simulink model "FSAC2021_V1_Running"  (R2014a)
settings: Solver=FixedStepDiscrete  StartTime=0.0  StopTime=inf  FixedStep=0.0005  RelTol=1e-3
model workspace (MAT data in the model file):
  MCOS : class17 (value not decoded)
  MCOS : class17 (value not decoded)
  MCOS : class17 (value not decoded)
  MCOS : class17 (value not decoded)
  MCOS : class17 (value not decoded)
  MCOS : class17 (value not decoded)
  MCOS : class17 (value not decoded)
  MCOS : class17 (value not decoded)
  MCOS : class17 (value not decoded)
  MCOS : class17 (value not decoded)
  MCOS : class17 (value not decoded)
  MCOS : class17 (value not decoded)
  MCOS : class17 (value not decoded)
  MCOS : class17 (value not decoded)
  MCOS : class17 (value not decoded)
  MCOS : class17 (value not decoded)
  MCOS : class17 (value not decoded)
  MCOS : class17 (value not decoded)
  MCOS : class17 (value not decoded)
  BUZZER_START = 1
  MCOS : class17 (value not decoded)
  MCOS : class17 (value not decoded)
  MCOS : class17 (value not decoded)
  MCOS : class17 (value not decoded)
  MCOS : class17 (value not decoded)
  MCOS : class17 (value not decoded)
  MCOS : class17 (value not decoded)
  MCOS : class17 (value not decoded)
  MCOS : class17 (value not decoded)
  MCOS : class17 (value not decoded)
  MCOS : class17 (value not decoded)
  MCOS : class17 (value not decoded)
  MCOS : class17 (value not decoded)
  MCOS : class17 (value not decoded)
  MCOS : class17 (value not decoded)
  MCOS : class17 (value not decoded)
  MCOS : class17 (value not decoded)
  MCOS : class17 (value not decoded)
  MCOS : class17 (value not decoded)
  MCOS : class17 (value not decoded)
  MCOS : class17 (value not decoded)
  MCOS : class17 (value not decoded)
  MCOS : class17 (value not decoded)
  MCOS : class17 (value not decoded)
  MCOS : class17 (value not decoded)
  MCOS : class17 (value not decoded)
  MCOS : class17 (value not decoded)
  MCOS : class17 (value not decoded)
  MCOS : class17 (value not decoded)
  MCOS : class17 (value not decoded)
  MCOS : class17 (value not decoded)
  MCOS : class17 (value not decoded)
  MCOS : class17 (value not decoded)
  MCOS : class17 (value not decoded)
  MCOS : class17 (value not decoded)
  MCOS : class17 (value not decoded)
  MCOS : class17 (value not decoded)
  MCOS : class17 (value not decoded)
  Brake = 11
  MCOS : class17 (value not decoded)
  MCOS : class17 (value not decoded)
  MCOS : class17 (value not decoded)
  MCOS : class17 (value not decoded)
  MCOS : class17 (value not decoded)
  MCOS : class17 (value not decoded)
  MCOS : class17 (value not decoded)
  MCOS : class17 (value not decoded)
  Sensor_Acc_b = 101.85
  Sensor_Acc_k = -0.0185
  Str_Sen_Orig_Angle = -341
  MCOS : class17 (value not decoded)
  Tire_D = 0.47
  T = 0.05
libraries: simulink x402, ec55xxlib x134
(part 11 of 17)

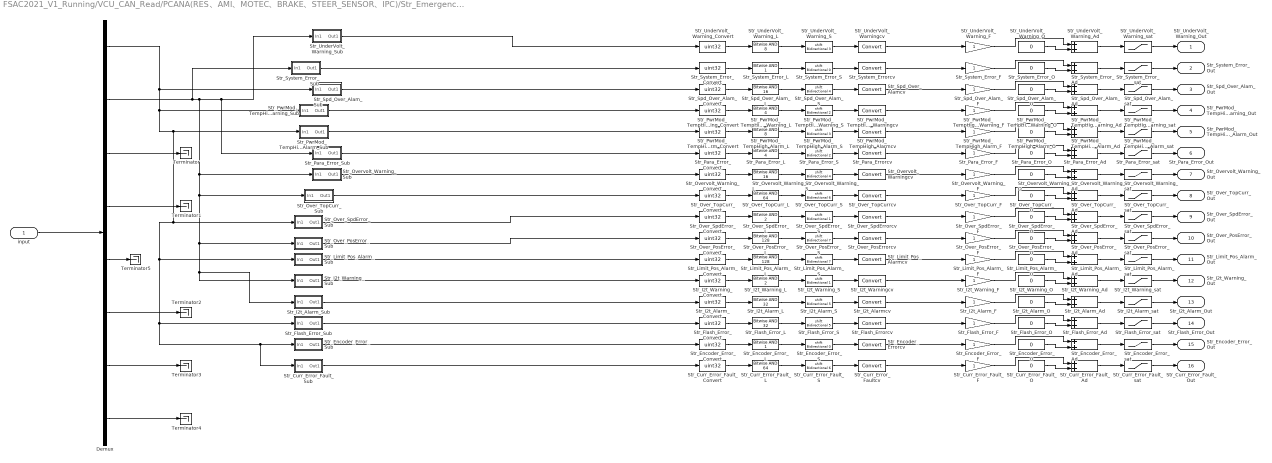
== system FSAC2021_V1_Running/VCU_CAN_Read/PCANA(RES、AMI、MOTEC、BRAKE、STEER_SENSOR、IPC)/Str_Emergency /MOTEC_EMERGENCY ==
  input : Inport
  Demux : Demux  Outputs=8
  Str_Curr_Error_Fault_Ad : Sum
  Str_Curr_Error_Fault_Convert : DataTypeConversion  OutDataTypeStr=uint32
  Str_Curr_Error_Fault_F : Gain
  Str_Curr_Error_Fault_L : simulink/Logic and Bit Operations/Bitwise Operator  logicop=AND  UseBitMask=on  BitMask=64  BitMaskRealWorld=Stored Integer
  Str_Curr_Error_Fault_O : Constant  Value=0  OutDataTypeStr=single
  Str_Curr_Error_Fault_S : ArithShift  BitShiftNumber=6
  Str_Curr_Error_Fault_Sub : Subsystem
  Str_Curr_Error_Fault_sat : Saturate  UpperLimit=1  LowerLimit=0
  Str_Curr_Error_Faultcv : DataTypeConversion
  Str_Encoder_Error_Ad : Sum
  Str_Encoder_Error_Convert : DataTypeConversion  OutDataTypeStr=uint32
  Str_Encoder_Error_F : Gain
  Str_Encoder_Error_L : simulink/Logic and Bit Operations/Bitwise Operator  logicop=AND  UseBitMask=on  BitMask=1  BitMaskRealWorld=Stored Integer
  Str_Encoder_Error_O : Constant  Value=0  OutDataTypeStr=single
  Str_Encoder_Error_S : ArithShift
  Str_Encoder_Error_Sub : Subsystem
  Str_Encoder_Error_sat : Saturate  UpperLimit=1  LowerLimit=0
  Str_Encoder_Errorcv : DataTypeConversion
  Str_Flash_Error_Ad : Sum
  Str_Flash_Error_Convert : DataTypeConversion  OutDataTypeStr=uint32
  Str_Flash_Error_F : Gain
  Str_Flash_Error_L : simulink/Logic and Bit Operations/Bitwise Operator  logicop=AND  UseBitMask=on  BitMask=32  BitMaskRealWorld=Stored Integer
  Str_Flash_Error_O : Constant  Value=0  OutDataTypeStr=single
  Str_Flash_Error_S : ArithShift  BitShiftNumber=5
  Str_Flash_Error_Sub : Subsystem
  Str_Flash_Error_sat : Saturate  UpperLimit=1  LowerLimit=0
  Str_Flash_Errorcv : DataTypeConversion
  Str_I2t_Alarm_Ad : Sum
  Str_I2t_Alarm_Convert : DataTypeConversion  OutDataTypeStr=uint32
  Str_I2t_Alarm_F : Gain
  Str_I2t_Alarm_L : simulink/Logic and Bit Operations/Bitwise Operator  logicop=AND  UseBitMask=on  BitMask=32  BitMaskRealWorld=Stored Integer
  Str_I2t_Alarm_O : Constant  Value=0  OutDataTypeStr=single
  Str_I2t_Alarm_S : ArithShift  BitShiftNumber=5
  Str_I2t_Alarm_Sub : Subsystem
  Str_I2t_Alarm_sat : Saturate  UpperLimit=1  LowerLimit=0
  Str_I2t_Alarmcv : DataTypeConversion
  Str_I2t_Warning_Ad : Sum
  Str_I2t_Warning_Convert : DataTypeConversion  OutDataTypeStr=uint32
  Str_I2t_Warning_F : Gain
  Str_I2t_Warning_L : simulink/Logic and Bit Operations/Bitwise Operator  logicop=AND  UseBitMask=on  BitMask=2  BitMaskRealWorld=Stored Integer
  Str_I2t_Warning_O : Constant  Value=0  OutDataTypeStr=single
  Str_I2t_Warning_S : ArithShift  BitShiftNumber=1
  Str_I2t_Warning_Sub : Subsystem
  Str_I2t_Warning_sat : Saturate  UpperLimit=1  LowerLimit=0
  Str_I2t_Warningcv : DataTypeConversion
  Str_Limit_Pos_Alarm_Ad : Sum
  Str_Limit_Pos_Alarm_Convert : DataTypeConversion  OutDataTypeStr=uint32
  Str_Limit_Pos_Alarm_F : Gain
  Str_Limit_Pos_Alarm_L : simulink/Logic and Bit Operations/Bitwise Operator  logicop=AND  UseBitMask=on  BitMask=128  BitMaskRealWorld=Stored Integer
  Str_Limit_Pos_Alarm_O : Constant  Value=0  OutDataTypeStr=single
  Str_Limit_Pos_Alarm_S : ArithShift  BitShiftNumber=7
  Str_Limit_Pos_Alarm_Sub : Subsystem
  Str_Limit_Pos_Alarm_sat : Saturate  UpperLimit=1  LowerLimit=0
  Str_Limit_Pos_Alarmcv : DataTypeConversion
  Str_Over_PosError_Ad : Sum
  Str_Over_PosError_Convert : DataTypeConversion  OutDataTypeStr=uint32
  Str_Over_PosError_F : Gain
  Str_Over_PosError_L : simulink/Logic and Bit Operations/Bitwise Operator  logicop=AND  UseBitMask=on  BitMask=128  BitMaskRealWorld=Stored Integer
  Str_Over_PosError_O : Constant  Value=0  OutDataTypeStr=single
  Str_Over_PosError_S : ArithShift  BitShiftNumber=7
  Str_Over_PosError_Sub : Subsystem
  Str_Over_PosError_sat : Saturate  UpperLimit=1  LowerLimit=0
  Str_Over_PosErrorcv : DataTypeConversion
  Str_Over_SpdError_Ad : Sum
  Str_Over_SpdError_Convert : DataTypeConversion  OutDataTypeStr=uint32
  Str_Over_SpdError_F : Gain
  Str_Over_SpdError_L : simulink/Logic and Bit Operations/Bitwise Operator  logicop=AND  UseBitMask=on  BitMask=2  BitMaskRealWorld=Stored Integer
  Str_Over_SpdError_O : Constant  Value=0  OutDataTypeStr=single
  Str_Over_SpdError_S : ArithShift  BitShiftNumber=1
  Str_Over_SpdError_Sub : Subsystem
  Str_Over_SpdError_sat : Saturate  UpperLimit=1  LowerLimit=0
  Str_Over_SpdErrorcv : DataTypeConversion
  Str_Over_TopCurr_Ad : Sum
  Str_Over_TopCurr_Convert : DataTypeConversion  OutDataTypeStr=uint32
  Str_Over_TopCurr_F : Gain
  Str_Over_TopCurr_L : simulink/Logic and Bit Operations/Bitwise Operator  logicop=AND  UseBitMask=on  BitMask=64  BitMaskRealWorld=Stored Integer
  Str_Over_TopCurr_O : Constant  Value=0  OutDataTypeStr=single
  Str_Over_TopCurr_S : ArithShift  BitShiftNumber=6
  Str_Over_TopCurr_Sub : Subsystem
  Str_Over_TopCurr_sat : Saturate  UpperLimit=1  LowerLimit=0
  Str_Over_TopCurrcv : DataTypeConversion
  Str_Overvolt_Warning_Ad : Sum
  Str_Overvolt_Warning_Convert : DataTypeConversion  OutDataTypeStr=uint32
  Str_Overvolt_Warning_F : Gain
  Str_Overvolt_Warning_L : simulink/Logic and Bit Operations/Bitwise Operator  logicop=AND  UseBitMask=on  BitMask=16  BitMaskRealWorld=Stored Integer
  Str_Overvolt_Warning_O : Constant  Value=0  OutDataTypeStr=single
  Str_Overvolt_Warning_S : ArithShift  BitShiftNumber=4
  Str_Overvolt_Warning_Sub : Subsystem
  Str_Overvolt_Warning_sat : Saturate  UpperLimit=1  LowerLimit=0
  Str_Overvolt_Warningcv : DataTypeConversion
  Str_Para_Error_Ad : Sum
  Str_Para_Error_Convert : DataTypeConversion  OutDataTypeStr=uint32
  Str_Para_Error_F : Gain
  Str_Para_Error_L : simulink/Logic and Bit Operations/Bitwise Operator  logicop=AND  UseBitMask=on  BitMask=4  BitMaskRealWorld=Stored Integer
  Str_Para_Error_O : Constant  Value=0  OutDataTypeStr=single
  Str_Para_Error_S : ArithShift  BitShiftNumber=2
  Str_Para_Error_Sub : Subsystem
  Str_Para_Error_sat : Saturate  UpperLimit=1  LowerLimit=0
  Str_Para_Errorcv : DataTypeConversion
  Str_PwrMod_TempHigh_Alarm_Ad : Sum
  Str_PwrMod_TempHigh_Alarm_Convert : DataTypeConversion  OutDataTypeStr=uint32
  Str_PwrMod_TempHigh_Alarm_F : Gain
  Str_PwrMod_TempHigh_Alarm_L : simulink/Logic and Bit Operations/Bitwise Operator  logicop=AND  UseBitMask=on  BitMask=8  BitMaskRealWorld=Stored Integer
  Str_PwrMod_TempHigh_Alarm_O : Constant  Value=0  OutDataTypeStr=single
  Str_PwrMod_TempHigh_Alarm_S : ArithShift  BitShiftNumber=3
  Str_PwrMod_TempHigh_Alarm_Sub : Subsystem
  Str_PwrMod_TempHigh_Alarm_sat : Saturate  UpperLimit=1  LowerLimit=0
  Str_PwrMod_TempHigh_Alarmcv : DataTypeConversion
  Str_PwrMod_TempHigh_Warning_Ad : Sum
  Str_PwrMod_TempHigh_Warning_Convert : DataTypeConversion  OutDataTypeStr=uint32
  Str_PwrMod_TempHigh_Warning_F : Gain
  Str_PwrMod_TempHigh_Warning_L : simulink/Logic and Bit Operations/Bitwise Operator  logicop=AND  UseBitMask=on  BitMask=4  BitMaskRealWorld=Stored Integer
  Str_PwrMod_TempHigh_Warning_O : Constant  Value=0  OutDataTypeStr=single
  Str_PwrMod_TempHigh_Warning_S : ArithShift  BitShiftNumber=2
  Str_PwrMod_TempHigh_Warning_Sub : Subsystem
  Str_PwrMod_TempHigh_Warning_sat : Saturate  UpperLimit=1  LowerLimit=0
  Str_PwrMod_TempHigh_Warningcv : DataTypeConversion
  Str_Spd_Over_Alam_Ad : Sum
  Str_Spd_Over_Alam_Convert : DataTypeConversion  OutDataTypeStr=uint32
  Str_Spd_Over_Alam_F : Gain
  Str_Spd_Over_Alam_L : simulink/Logic and Bit Operations/Bitwise Operator  logicop=AND  UseBitMask=on  BitMask=16  BitMaskRealWorld=Stored Integer
  Str_Spd_Over_Alam_O : Constant  Value=0  OutDataTypeStr=single
  Str_Spd_Over_Alam_S : ArithShift  BitShiftNumber=4
  Str_Spd_Over_Alam_Sub : Subsystem
  Str_Spd_Over_Alam_sat : Saturate  UpperLimit=1  LowerLimit=0
  Str_Spd_Over_Alamcv : DataTypeConversion
  Str_System_Error_Ad : Sum
  Str_System_Error_Convert : DataTypeConversion  OutDataTypeStr=uint32
  Str_System_Error_F : Gain
  Str_System_Error_L : simulink/Logic and Bit Operations/Bitwise Operator  logicop=AND  UseBitMask=on  BitMask=1  BitMaskRealWorld=Stored Integer
  Str_System_Error_O : Constant  Value=0  OutDataTypeStr=single
  Str_System_Error_S : ArithShift
  Str_System_Error_Sub : Subsystem
  Str_System_Error_sat : Saturate  UpperLimit=1  LowerLimit=0
  Str_System_Errorcv : DataTypeConversion
  Str_UnderVolt_Warning_Ad : Sum
  Str_UnderVolt_Warning_Convert : DataTypeConversion  OutDataTypeStr=uint32
  Str_UnderVolt_Warning_F : Gain
  Str_UnderVolt_Warning_L : simulink/Logic and Bit Operations/Bitwise Operator  logicop=AND  UseBitMask=on  BitMask=8  BitMaskRealWorld=Stored Integer
  Str_UnderVolt_Warning_O : Constant  Value=0  OutDataTypeStr=single
  Str_UnderVolt_Warning_S : ArithShift  BitShiftNumber=3
  Str_UnderVolt_Warning_Sub : Subsystem
  Str_UnderVolt_Warning_sat : Saturate  UpperLimit=1  LowerLimit=0
  Str_UnderVolt_Warningcv : DataTypeConversion
  Terminator{,1..5} (6 alike) : Terminator
  Str_UnderVolt_Warning_Out : Outport
  Str_System_Error_Out : Outport  Port=2
  Str_Spd_Over_Alam_Out : Outport  Port=3
  Str_PwrMod_TempHigh_Warning_Out : Outport  Port=4
  Str_PwrMod_TempHigh_Alarm_Out : Outport  Port=5
  Str_Para_Error_Out : Outport  Port=6
  Str_Overvolt_Warning_Out : Outport  Port=7
  Str_Over_TopCurr_Out : Outport  Port=8
  Str_Over_SpdError_Out : Outport  Port=9
  Str_Over_PosError_Out : Outport  Port=10
  Str_Limit_Pos_Alarm_Out : Outport  Port=11
  Str_I2t_Warning_Out : Outport  Port=12
  Str_I2t_Alarm_Out : Outport  Port=13
  Str_Flash_Error_Out : Outport  Port=14
  Str_Encoder_Error_Out : Outport  Port=15
  Str_Curr_Error_Fault_Out : Outport  Port=16
  wires:
  Str_UnderVolt_Warning_F/1 -> Str_UnderVolt_Warning_Ad/1
  Str_UnderVolt_Warning_O/1 -> Str_UnderVolt_Warning_Ad/2
  Str_UnderVolt_Warning_Ad/1 -> Str_UnderVolt_Warning_sat/1
  Str_UnderVolt_Warning_sat/1 -> Str_UnderVolt_Warning_Out/1
  Demux/2 -> Str_Para_Error_Sub/1(In1), Str_UnderVolt_Warning_Sub/1(In1), Str_I2t_Warning_Sub/1(In1), Str_I2t_Alarm_Sub/1(In1), Str_Over_PosError_Sub/1(In1), Str_Over_TopCurr_Sub/1(In1), Str_Overvolt_Warning_Sub/1(In1), Str_System_Error_Sub/1(In1)
  Str_UnderVolt_Warning_Sub/1(Out1) -> Str_UnderVolt_Warning_Convert/1
  Str_UnderVolt_Warning_Convert/1 -> Str_UnderVolt_Warning_L/1
  Str_UnderVolt_Warning_L/1 -> Str_UnderVolt_Warning_S/1
  Str_UnderVolt_Warning_S/1 -> Str_UnderVolt_Warningcv/1
  Str_UnderVolt_Warningcv/1 -> Str_UnderVolt_Warning_F/1
  Str_System_Error_F/1 -> Str_System_Error_Ad/1
  Str_System_Error_O/1 -> Str_System_Error_Ad/2
  Str_System_Error_Ad/1 -> Str_System_Error_sat/1
  Str_System_Error_sat/1 -> Str_System_Error_Out/1
  Str_System_Error_Sub/1(Out1) -> Str_System_Error_Convert/1
  Str_System_Error_Convert/1 -> Str_System_Error_L/1
  Str_System_Error_L/1 -> Str_System_Error_S/1
  Str_System_Error_S/1 -> Str_System_Errorcv/1
  Str_System_Errorcv/1 -> Str_System_Error_F/1
  Str_Spd_Over_Alam_F/1 -> Str_Spd_Over_Alam_Ad/1
  Str_Spd_Over_Alam_O/1 -> Str_Spd_Over_Alam_Ad/2
  Str_Spd_Over_Alam_Ad/1 -> Str_Spd_Over_Alam_sat/1
  Str_Spd_Over_Alam_sat/1 -> Str_Spd_Over_Alam_Out/1
  Demux/1 -> Str_Encoder_Error_Sub/1(In1), Str_Curr_Error_Fault_Sub/1(In1), Str_Flash_Error_Sub/1(In1), Str_Limit_Pos_Alarm_Sub/1(In1), Str_Over_SpdError_Sub/1(In1), Str_PwrMod_TempHigh_Alarm_Sub/1(In1), Str_PwrMod_TempHigh_Warning_Sub/1(In1), Str_Spd_Over_Alam_Sub/1(In1)
  Str_Spd_Over_Alam_Sub/1(Out1) -> Str_Spd_Over_Alam_Convert/1
  Str_Spd_Over_Alam_Convert/1 -> Str_Spd_Over_Alam_L/1
  Str_Spd_Over_Alam_L/1 -> Str_Spd_Over_Alam_S/1
  Str_Spd_Over_Alam_S/1 -> Str_Spd_Over_Alamcv/1
  Str_Spd_Over_Alamcv/1 -> Str_Spd_Over_Alam_F/1
  Str_PwrMod_TempHigh_Warning_F/1 -> Str_PwrMod_TempHigh_Warning_Ad/1
  Str_PwrMod_TempHigh_Warning_O/1 -> Str_PwrMod_TempHigh_Warning_Ad/2
  Str_PwrMod_TempHigh_Warning_Ad/1 -> Str_PwrMod_TempHigh_Warning_sat/1
  Str_PwrMod_TempHigh_Warning_sat/1 -> Str_PwrMod_TempHigh_Warning_Out/1
  Str_PwrMod_TempHigh_Warning_Sub/1(Out1) -> Str_PwrMod_TempHigh_Warning_Convert/1
  Str_PwrMod_TempHigh_Warning_Convert/1 -> Str_PwrMod_TempHigh_Warning_L/1
  Str_PwrMod_TempHigh_Warning_L/1 -> Str_PwrMod_TempHigh_Warning_S/1
  Str_PwrMod_TempHigh_Warning_S/1 -> Str_PwrMod_TempHigh_Warningcv/1
  Str_PwrMod_TempHigh_Warningcv/1 -> Str_PwrMod_TempHigh_Warning_F/1
  Str_PwrMod_TempHigh_Alarm_F/1 -> Str_PwrMod_TempHigh_Alarm_Ad/1
  Str_PwrMod_TempHigh_Alarm_O/1 -> Str_PwrMod_TempHigh_Alarm_Ad/2
  Str_PwrMod_TempHigh_Alarm_Ad/1 -> Str_PwrMod_TempHigh_Alarm_sat/1
  Str_PwrMod_TempHigh_Alarm_sat/1 -> Str_PwrMod_TempHigh_Alarm_Out/1
  Str_PwrMod_TempHigh_Alarm_Sub/1(Out1) -> Str_PwrMod_TempHigh_Alarm_Convert/1
  Str_PwrMod_TempHigh_Alarm_Convert/1 -> Str_PwrMod_TempHigh_Alarm_L/1
  Str_PwrMod_TempHigh_Alarm_L/1 -> Str_PwrMod_TempHigh_Alarm_S/1
  Str_PwrMod_TempHigh_Alarm_S/1 -> Str_PwrMod_TempHigh_Alarmcv/1
  Str_PwrMod_TempHigh_Alarmcv/1 -> Str_PwrMod_TempHigh_Alarm_F/1
  Str_Para_Error_F/1 -> Str_Para_Error_Ad/1
  Str_Para_Error_O/1 -> Str_Para_Error_Ad/2
  Str_Para_Error_Ad/1 -> Str_Para_Error_sat/1
  Str_Para_Error_sat/1 -> Str_Para_Error_Out/1
  Str_Para_Error_Sub/1(Out1) -> Str_Para_Error_Convert/1
  Str_Para_Error_Convert/1 -> Str_Para_Error_L/1
  Str_Para_Error_L/1 -> Str_Para_Error_S/1
  Str_Para_Error_S/1 -> Str_Para_Errorcv/1
  Str_Para_Errorcv/1 -> Str_Para_Error_F/1
  Str_Overvolt_Warning_F/1 -> Str_Overvolt_Warning_Ad/1
  Str_Overvolt_Warning_O/1 -> Str_Overvolt_Warning_Ad/2
  Str_Overvolt_Warning_Ad/1 -> Str_Overvolt_Warning_sat/1
  Str_Overvolt_Warning_sat/1 -> Str_Overvolt_Warning_Out/1
  Str_Overvolt_Warning_Sub/1(Out1) -> Str_Overvolt_Warning_Convert/1
  Str_Overvolt_Warning_Convert/1 -> Str_Overvolt_Warning_L/1
  Str_Overvolt_Warning_L/1 -> Str_Overvolt_Warning_S/1
  Str_Overvolt_Warning_S/1 -> Str_Overvolt_Warningcv/1
  Str_Overvolt_Warningcv/1 -> Str_Overvolt_Warning_F/1
  Str_Over_TopCurr_F/1 -> Str_Over_TopCurr_Ad/1
  Str_Over_TopCurr_O/1 -> Str_Over_TopCurr_Ad/2
  Str_Over_TopCurr_Ad/1 -> Str_Over_TopCurr_sat/1
  Str_Over_TopCurr_sat/1 -> Str_Over_TopCurr_Out/1
  Str_Over_TopCurr_Sub/1(Out1) -> Str_Over_TopCurr_Convert/1
  Str_Over_TopCurr_Convert/1 -> Str_Over_TopCurr_L/1
  Str_Over_TopCurr_L/1 -> Str_Over_TopCurr_S/1
  Str_Over_TopCurr_S/1 -> Str_Over_TopCurrcv/1
  Str_Over_TopCurrcv/1 -> Str_Over_TopCurr_F/1
  Str_Over_SpdError_F/1 -> Str_Over_SpdError_Ad/1
  Str_Over_SpdError_O/1 -> Str_Over_SpdError_Ad/2
  Str_Over_SpdError_Ad/1 -> Str_Over_SpdError_sat/1
  Str_Over_SpdError_sat/1 -> Str_Over_SpdError_Out/1
  Str_Over_SpdError_Sub/1(Out1) -> Str_Over_SpdError_Convert/1
  Str_Over_SpdError_Convert/1 -> Str_Over_SpdError_L/1
  Str_Over_SpdError_L/1 -> Str_Over_SpdError_S/1
  Str_Over_SpdError_S/1 -> Str_Over_SpdErrorcv/1
  Str_Over_SpdErrorcv/1 -> Str_Over_SpdError_F/1
  Str_Over_PosError_F/1 -> Str_Over_PosError_Ad/1
  Str_Over_PosError_O/1 -> Str_Over_PosError_Ad/2
  Str_Over_PosError_Ad/1 -> Str_Over_PosError_sat/1
  Str_Over_PosError_sat/1 -> Str_Over_PosError_Out/1
  Str_Over_PosError_Sub/1(Out1) -> Str_Over_PosError_Convert/1
  Str_Over_PosError_Convert/1 -> Str_Over_PosError_L/1
  Str_Over_PosError_L/1 -> Str_Over_PosError_S/1
  Str_Over_PosError_S/1 -> Str_Over_PosErrorcv/1
  Str_Over_PosErrorcv/1 -> Str_Over_PosError_F/1
  Str_Limit_Pos_Alarm_F/1 -> Str_Limit_Pos_Alarm_Ad/1
  Str_Limit_Pos_Alarm_O/1 -> Str_Limit_Pos_Alarm_Ad/2
  Str_Limit_Pos_Alarm_Ad/1 -> Str_Limit_Pos_Alarm_sat/1
  Str_Limit_Pos_Alarm_sat/1 -> Str_Limit_Pos_Alarm_Out/1
  Str_Limit_Pos_Alarm_Sub/1(Out1) -> Str_Limit_Pos_Alarm_Convert/1
  Str_Limit_Pos_Alarm_Convert/1 -> Str_Limit_Pos_Alarm_L/1
  Str_Limit_Pos_Alarm_L/1 -> Str_Limit_Pos_Alarm_S/1
  Str_Limit_Pos_Alarm_S/1 -> Str_Limit_Pos_Alarmcv/1
  Str_Limit_Pos_Alarmcv/1 -> Str_Limit_Pos_Alarm_F/1
  Str_I2t_Warning_F/1 -> Str_I2t_Warning_Ad/1
  Str_I2t_Warning_O/1 -> Str_I2t_Warning_Ad/2
  Str_I2t_Warning_Ad/1 -> Str_I2t_Warning_sat/1
  Str_I2t_Warning_sat/1 -> Str_I2t_Warning_Out/1
  Str_I2t_Warning_Sub/1(Out1) -> Str_I2t_Warning_Convert/1
  Str_I2t_Warning_Convert/1 -> Str_I2t_Warning_L/1
  Str_I2t_Warning_L/1 -> Str_I2t_Warning_S/1
  Str_I2t_Warning_S/1 -> Str_I2t_Warningcv/1
  Str_I2t_Warningcv/1 -> Str_I2t_Warning_F/1
  Str_I2t_Alarm_F/1 -> Str_I2t_Alarm_Ad/1
  Str_I2t_Alarm_O/1 -> Str_I2t_Alarm_Ad/2
  Str_I2t_Alarm_Ad/1 -> Str_I2t_Alarm_sat/1
  Str_I2t_Alarm_sat/1 -> Str_I2t_Alarm_Out/1
  Str_I2t_Alarm_Sub/1(Out1) -> Str_I2t_Alarm_Convert/1
  Str_I2t_Alarm_Convert/1 -> Str_I2t_Alarm_L/1
  Str_I2t_Alarm_L/1 -> Str_I2t_Alarm_S/1
  Str_I2t_Alarm_S/1 -> Str_I2t_Alarmcv/1
  Str_I2t_Alarmcv/1 -> Str_I2t_Alarm_F/1
  Str_Flash_Error_F/1 -> Str_Flash_Error_Ad/1
  Str_Flash_Error_O/1 -> Str_Flash_Error_Ad/2
  Str_Flash_Error_Ad/1 -> Str_Flash_Error_sat/1
  Str_Flash_Error_sat/1 -> Str_Flash_Error_Out/1
  Str_Flash_Error_Sub/1(Out1) -> Str_Flash_Error_Convert/1
  Str_Flash_Error_Convert/1 -> Str_Flash_Error_L/1
  Str_Flash_Error_L/1 -> Str_Flash_Error_S/1
  Str_Flash_Error_S/1 -> Str_Flash_Errorcv/1
  Str_Flash_Errorcv/1 -> Str_Flash_Error_F/1
  Str_Encoder_Error_F/1 -> Str_Encoder_Error_Ad/1
  Str_Encoder_Error_O/1 -> Str_Encoder_Error_Ad/2
  Str_Encoder_Error_Ad/1 -> Str_Encoder_Error_sat/1
  Str_Encoder_Error_sat/1 -> Str_Encoder_Error_Out/1
  Str_Encoder_Error_Sub/1(Out1) -> Str_Encoder_Error_Convert/1
  Str_Encoder_Error_Convert/1 -> Str_Encoder_Error_L/1
  Str_Encoder_Error_L/1 -> Str_Encoder_Error_S/1
  Str_Encoder_Error_S/1 -> Str_Encoder_Errorcv/1
  Str_Encoder_Errorcv/1 -> Str_Encoder_Error_F/1
  Str_Curr_Error_Fault_F/1 -> Str_Curr_Error_Fault_Ad/1
  Str_Curr_Error_Fault_O/1 -> Str_Curr_Error_Fault_Ad/2
  Str_Curr_Error_Fault_Ad/1 -> Str_Curr_Error_Fault_sat/1
  Str_Curr_Error_Fault_sat/1 -> Str_Curr_Error_Fault_Out/1
  Str_Curr_Error_Fault_Sub/1(Out1) -> Str_Curr_Error_Fault_Convert/1
  Str_Curr_Error_Fault_Convert/1 -> Str_Curr_Error_Fault_L/1
  Str_Curr_Error_Fault_L/1 -> Str_Curr_Error_Fault_S/1
  Str_Curr_Error_Fault_S/1 -> Str_Curr_Error_Faultcv/1
  Str_Curr_Error_Faultcv/1 -> Str_Curr_Error_Fault_F/1
  input/1 -> Demux/1
  Demux/3 -> Terminator/1
  Demux/4 -> Terminator1/1
  Demux/6 -> Terminator2/1
  Demux/7 -> Terminator3/1
  Demux/8 -> Terminator4/1
  Demux/5 -> Terminator5/1

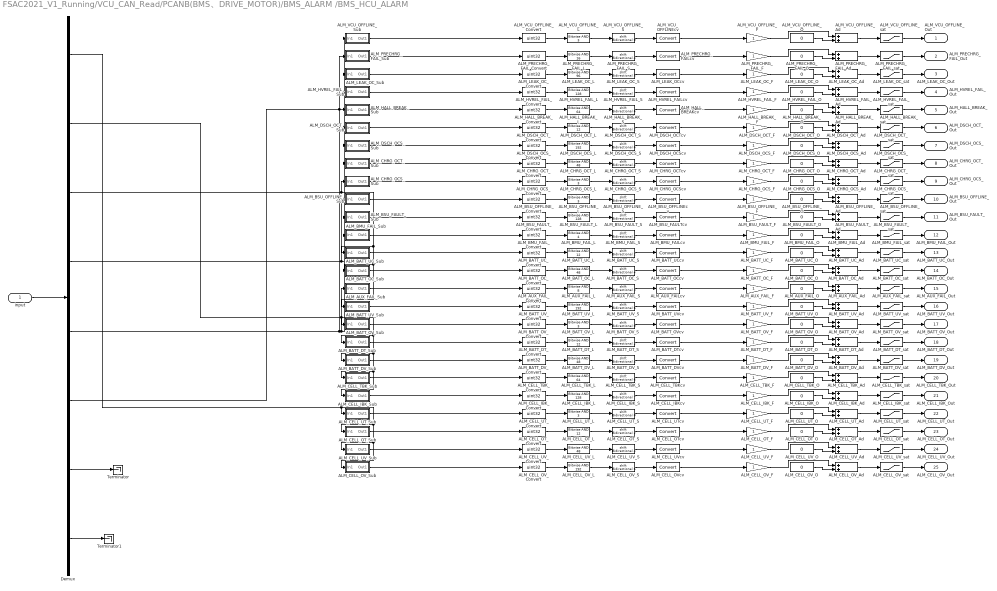
== system FSAC2021_V1_Running/VCU_CAN_Read/PCANB(BMS、DRIVE_MOTOR)/BMS_ALARM /BMS_HCU_ALARM ==
  input : Inport
  ALM_AUX_FAIL_Ad : Sum
  ALM_AUX_FAIL_Convert : DataTypeConversion  OutDataTypeStr=uint32
  ALM_AUX_FAIL_F : Gain
  ALM_AUX_FAIL_L : simulink/Logic and Bit Operations/Bitwise Operator  logicop=AND  UseBitMask=on  BitMask=8  BitMaskRealWorld=Stored Integer
  ALM_AUX_FAIL_O : Constant  Value=0  OutDataTypeStr=single
  ALM_AUX_FAIL_S : ArithShift  BitShiftNumber=3
  ALM_AUX_FAIL_Sub : Subsystem
  ALM_AUX_FAIL_sat : Saturate  UpperLimit=1  LowerLimit=0
  ALM_AUX_FAILcv : DataTypeConversion
  ALM_BATT_DT_Ad : Sum
  ALM_BATT_DT_Convert : DataTypeConversion  OutDataTypeStr=uint32
  ALM_BATT_DT_F : Gain
  ALM_BATT_DT_L : simulink/Logic and Bit Operations/Bitwise Operator  logicop=AND  UseBitMask=on  BitMask=12  BitMaskRealWorld=Stored Integer
  ALM_BATT_DT_O : Constant  Value=0  OutDataTypeStr=single
  ALM_BATT_DT_S : ArithShift  BitShiftNumber=2
  ALM_BATT_DT_Sub : Subsystem
  ALM_BATT_DT_sat : Saturate  UpperLimit=3  LowerLimit=0
  ALM_BATT_DTcv : DataTypeConversion
  ALM_BATT_DV_Ad : Sum
  ALM_BATT_DV_Convert : DataTypeConversion  OutDataTypeStr=uint32
  ALM_BATT_DV_F : Gain
  ALM_BATT_DV_L : simulink/Logic and Bit Operations/Bitwise Operator  logicop=AND  UseBitMask=on  BitMask=48  BitMaskRealWorld=Stored Integer
  ALM_BATT_DV_O : Constant  Value=0  OutDataTypeStr=single
  ALM_BATT_DV_S : ArithShift  BitShiftNumber=4
  ALM_BATT_DV_Sub : Subsystem
  ALM_BATT_DV_sat : Saturate  UpperLimit=3  LowerLimit=0
  ALM_BATT_DVcv : DataTypeConversion
  ALM_BATT_OC_Ad : Sum
  ALM_BATT_OC_Convert : DataTypeConversion  OutDataTypeStr=uint32
  ALM_BATT_OC_F : Gain
  ALM_BATT_OC_L : simulink/Logic and Bit Operations/Bitwise Operator  logicop=AND  UseBitMask=on  BitMask=48  BitMaskRealWorld=Stored Integer
  ALM_BATT_OC_O : Constant  Value=0  OutDataTypeStr=single
  ALM_BATT_OC_S : ArithShift  BitShiftNumber=4
  ALM_BATT_OC_Sub : Subsystem
  ALM_BATT_OC_sat : Saturate  UpperLimit=3  LowerLimit=0
  ALM_BATT_OCcv : DataTypeConversion
  ALM_BATT_OV_Ad : Sum
  ALM_BATT_OV_Convert : DataTypeConversion  OutDataTypeStr=uint32
  ALM_BATT_OV_F : Gain
  ALM_BATT_OV_L : simulink/Logic and Bit Operations/Bitwise Operator  logicop=AND  UseBitMask=on  BitMask=3  BitMaskRealWorld=Stored Integer
  ALM_BATT_OV_O : Constant  Value=0  OutDataTypeStr=single
  ALM_BATT_OV_S : ArithShift
  ALM_BATT_OV_Sub : Subsystem
  ALM_BATT_OV_sat : Saturate  UpperLimit=3  LowerLimit=0
  ALM_BATT_OVcv : DataTypeConversion
  ALM_BATT_UC_Ad : Sum
  ALM_BATT_UC_Convert : DataTypeConversion  OutDataTypeStr=uint32
  ALM_BATT_UC_F : Gain
  ALM_BATT_UC_L : simulink/Logic and Bit Operations/Bitwise Operator  logicop=AND  UseBitMask=on  BitMask=12  BitMaskRealWorld=Stored Integer
  ALM_BATT_UC_O : Constant  Value=0  OutDataTypeStr=single
  ALM_BATT_UC_S : ArithShift  BitShiftNumber=2
  ALM_BATT_UC_Sub : Subsystem
  ALM_BATT_UC_sat : Saturate  UpperLimit=3  LowerLimit=0
  ALM_BATT_UCcv : DataTypeConversion
  ALM_BATT_UV_Ad : Sum
  ALM_BATT_UV_Convert : DataTypeConversion  OutDataTypeStr=uint32
  ALM_BATT_UV_F : Gain
  ALM_BATT_UV_L : simulink/Logic and Bit Operations/Bitwise Operator  logicop=AND  UseBitMask=on  BitMask=192  BitMaskRealWorld=Stored Integer
  ALM_BATT_UV_O : Constant  Value=0  OutDataTypeStr=single
  ALM_BATT_UV_S : ArithShift  BitShiftNumber=6
  ALM_BATT_UV_Sub : Subsystem
  ALM_BATT_UV_sat : Saturate  UpperLimit=3  LowerLimit=0
  ALM_BATT_UVcv : DataTypeConversion
  ALM_BMU_FAIL_Ad : Sum
  ALM_BMU_FAIL_Convert : DataTypeConversion  OutDataTypeStr=uint32
  ALM_BMU_FAIL_F : Gain
  ALM_BMU_FAIL_L : simulink/Logic and Bit Operations/Bitwise Operator  logicop=AND  UseBitMask=on  BitMask=4  BitMaskRealWorld=Stored Integer
  ALM_BMU_FAIL_O : Constant  Value=0  OutDataTypeStr=single
  ALM_BMU_FAIL_S : ArithShift  BitShiftNumber=2
  ALM_BMU_FAIL_Sub : Subsystem
  ALM_BMU_FAIL_sat : Saturate  UpperLimit=1  LowerLimit=0
  ALM_BMU_FAILcv : DataTypeConversion
  ALM_BSU_FAULT_Ad : Sum
  ALM_BSU_FAULT_Convert : DataTypeConversion  OutDataTypeStr=uint32
  ALM_BSU_FAULT_F : Gain
  ALM_BSU_FAULT_L : simulink/Logic and Bit Operations/Bitwise Operator  logicop=AND  UseBitMask=on  BitMask=128  BitMaskRealWorld=Stored Integer
  ALM_BSU_FAULT_O : Constant  Value=0  OutDataTypeStr=single
  ALM_BSU_FAULT_S : ArithShift  BitShiftNumber=7
  ALM_BSU_FAULT_Sub : Subsystem
  ALM_BSU_FAULT_sat : Saturate  UpperLimit=1  LowerLimit=0
  ALM_BSU_FAULTcv : DataTypeConversion
  ALM_BSU_OFFLINE_Ad : Sum
  ALM_BSU_OFFLINE_Convert : DataTypeConversion  OutDataTypeStr=uint32
  ALM_BSU_OFFLINE_F : Gain
  ALM_BSU_OFFLINE_L : simulink/Logic and Bit Operations/Bitwise Operator  logicop=AND  UseBitMask=on  BitMask=3  BitMaskRealWorld=Stored Integer
  ALM_BSU_OFFLINE_O : Constant  Value=0  OutDataTypeStr=single
  ALM_BSU_OFFLINE_S : ArithShift
  ALM_BSU_OFFLINE_Sub : Subsystem
  ALM_BSU_OFFLINE_sat : Saturate  UpperLimit=3  LowerLimit=0
  ALM_BSU_OFFLINEcv : DataTypeConversion
  ALM_CELL_IBK_Ad : Sum
  ALM_CELL_IBK_Convert : DataTypeConversion  OutDataTypeStr=uint32
  ALM_CELL_IBK_F : Gain
  ALM_CELL_IBK_L : simulink/Logic and Bit Operations/Bitwise Operator  logicop=AND  UseBitMask=on  BitMask=128  BitMaskRealWorld=Stored Integer
  ALM_CELL_IBK_O : Constant  Value=0  OutDataTypeStr=single
  ALM_CELL_IBK_S : ArithShift  BitShiftNumber=7
  ALM_CELL_IBK_Sub : Subsystem
  ALM_CELL_IBK_sat : Saturate  UpperLimit=1  LowerLimit=0
  ALM_CELL_IBKcv : DataTypeConversion
  ALM_CELL_OT_Ad : Sum
  ALM_CELL_OT_Convert : DataTypeConversion  OutDataTypeStr=uint32
  ALM_CELL_OT_F : Gain
  ALM_CELL_OT_L : simulink/Logic and Bit Operations/Bitwise Operator  logicop=AND  UseBitMask=on  BitMask=12  BitMaskRealWorld=Stored Integer
  ALM_CELL_OT_O : Constant  Value=0  OutDataTypeStr=single
  ALM_CELL_OT_S : ArithShift  BitShiftNumber=2
  ALM_CELL_OT_Sub : Subsystem
  ALM_CELL_OT_sat : Saturate  UpperLimit=3  LowerLimit=0
  ALM_CELL_OTcv : DataTypeConversion
  ALM_CELL_OV_Ad : Sum
  ALM_CELL_OV_Convert : DataTypeConversion  OutDataTypeStr=uint32
  ALM_CELL_OV_F : Gain
  ALM_CELL_OV_L : simulink/Logic and Bit Operations/Bitwise Operator  logicop=AND  UseBitMask=on  BitMask=192  BitMaskRealWorld=Stored Integer
  ALM_CELL_OV_O : Constant  Value=0  OutDataTypeStr=single
  ALM_CELL_OV_S : ArithShift  BitShiftNumber=6
  ALM_CELL_OV_Sub : Subsystem
  ALM_CELL_OV_sat : Saturate  UpperLimit=3  LowerLimit=0
  ALM_CELL_OVcv : DataTypeConversion
  ALM_CELL_TBK_Ad : Sum
  ALM_CELL_TBK_Convert : DataTypeConversion  OutDataTypeStr=uint32
  ALM_CELL_TBK_F : Gain
  ALM_CELL_TBK_L : simulink/Logic and Bit Operations/Bitwise Operator  logicop=AND  UseBitMask=on  BitMask=64  BitMaskRealWorld=Stored Integer
  ALM_CELL_TBK_O : Constant  Value=0  OutDataTypeStr=single
  ALM_CELL_TBK_S : ArithShift  BitShiftNumber=6
  ALM_CELL_TBK_Sub : Subsystem
  ALM_CELL_TBK_sat : Saturate  UpperLimit=1  LowerLimit=0
  ALM_CELL_TBKcv : DataTypeConversion
  ALM_CELL_UT_Ad : Sum
  ALM_CELL_UT_Convert : DataTypeConversion  OutDataTypeStr=uint32
  ALM_CELL_UT_F : Gain
  ALM_CELL_UT_L : simulink/Logic and Bit Operations/Bitwise Operator  logicop=AND  UseBitMask=on  BitMask=3  BitMaskRealWorld=Stored Integer
  ALM_CELL_UT_O : Constant  Value=0  OutDataTypeStr=single
  ALM_CELL_UT_S : ArithShift
  ALM_CELL_UT_Sub : Subsystem
  ALM_CELL_UT_sat : Saturate  UpperLimit=3  LowerLimit=0
  ALM_CELL_UTcv : DataTypeConversion
  ALM_CELL_UV_Ad : Sum
  ALM_CELL_UV_Convert : DataTypeConversion  OutDataTypeStr=uint32
  ALM_CELL_UV_F : Gain
  ALM_CELL_UV_L : simulink/Logic and Bit Operations/Bitwise Operator  logicop=AND  UseBitMask=on  BitMask=48  BitMaskRealWorld=Stored Integer
  ALM_CELL_UV_O : Constant  Value=0  OutDataTypeStr=single
  ALM_CELL_UV_S : ArithShift  BitShiftNumber=4
  ALM_CELL_UV_Sub : Subsystem
  ALM_CELL_UV_sat : Saturate  UpperLimit=3  LowerLimit=0
  ALM_CELL_UVcv : DataTypeConversion
  ALM_CHRG_OCS_Ad : Sum
  ALM_CHRG_OCS_Convert : DataTypeConversion  OutDataTypeStr=uint32
  ALM_CHRG_OCS_F : Gain
  ALM_CHRG_OCS_L : simulink/Logic and Bit Operations/Bitwise Operator  logicop=AND  UseBitMask=on  BitMask=3  BitMaskRealWorld=Stored Integer
  ALM_CHRG_OCS_O : Constant  Value=0  OutDataTypeStr=single
  ALM_CHRG_OCS_S : ArithShift
  ALM_CHRG_OCS_Sub : Subsystem
  ALM_CHRG_OCS_sat : Saturate  UpperLimit=3  LowerLimit=0
  ALM_CHRG_OCScv : DataTypeConversion
  ALM_CHRG_OCT_Ad : Sum
  ALM_CHRG_OCT_Convert : DataTypeConversion  OutDataTypeStr=uint32
  ALM_CHRG_OCT_F : Gain
  ALM_CHRG_OCT_L : simulink/Logic and Bit Operations/Bitwise Operator  logicop=AND  UseBitMask=on  BitMask=48  BitMaskRealWorld=Stored Integer
  ALM_CHRG_OCT_O : Constant  Value=0  OutDataTypeStr=single
  ALM_CHRG_OCT_S : ArithShift  BitShiftNumber=4
  ALM_CHRG_OCT_Sub : Subsystem
  ALM_CHRG_OCT_sat : Saturate  UpperLimit=3  LowerLimit=0
  ALM_CHRG_OCTcv : DataTypeConversion
  ALM_DSCH_OCS_Ad : Sum
  ALM_DSCH_OCS_Convert : DataTypeConversion  OutDataTypeStr=uint32
  ALM_DSCH_OCS_F : Gain
  ALM_DSCH_OCS_L : simulink/Logic and Bit Operations/Bitwise Operator  logicop=AND  UseBitMask=on  BitMask=192  BitMaskRealWorld=Stored Integer
  ALM_DSCH_OCS_O : Constant  Value=0  OutDataTypeStr=single
  ALM_DSCH_OCS_S : ArithShift  BitShiftNumber=6
  ALM_DSCH_OCS_Sub : Subsystem
  ALM_DSCH_OCS_sat : Saturate  UpperLimit=3  LowerLimit=0
  ALM_DSCH_OCScv : DataTypeConversion
  ALM_DSCH_OCT_Ad : Sum
  ALM_DSCH_OCT_Convert : DataTypeConversion  OutDataTypeStr=uint32
  ALM_DSCH_OCT_F : Gain
  ALM_DSCH_OCT_L : simulink/Logic and Bit Operations/Bitwise Operator  logicop=AND  UseBitMask=on  BitMask=12  BitMaskRealWorld=Stored Integer
  ALM_DSCH_OCT_O : Constant  Value=0  OutDataTypeStr=single
  ALM_DSCH_OCT_S : ArithShift  BitShiftNumber=2
  ALM_DSCH_OCT_Sub : Subsystem
  ALM_DSCH_OCT_sat : Saturate  UpperLimit=3  LowerLimit=0
  ALM_DSCH_OCTcv : DataTypeConversion
  ALM_HALL_BREAK_Ad : Sum
  ALM_HALL_BREAK_Convert : DataTypeConversion  OutDataTypeStr=uint32
  ALM_HALL_BREAK_F : Gain
  ALM_HALL_BREAK_L : simulink/Logic and Bit Operations/Bitwise Operator  logicop=AND  UseBitMask=on  BitMask=64  BitMaskRealWorld=Stored Integer
  ALM_HALL_BREAK_O : Constant  Value=0  OutDataTypeStr=single
  ALM_HALL_BREAK_S : ArithShift  BitShiftNumber=6
  ALM_HALL_BREAK_Sub : Subsystem
  ALM_HALL_BREAK_sat : Saturate  UpperLimit=1  LowerLimit=0
  ALM_HALL_BREAKcv : DataTypeConversion
  ALM_HVREL_FAIL_Ad : Sum
  ALM_HVREL_FAIL_Convert : DataTypeConversion  OutDataTypeStr=uint32
  ALM_HVREL_FAIL_F : Gain
  ALM_HVREL_FAIL_L : simulink/Logic and Bit Operations/Bitwise Operator  logicop=AND  UseBitMask=on  BitMask=128  BitMaskRealWorld=Stored Integer
  ALM_HVREL_FAIL_O : Constant  Value=0  OutDataTypeStr=single
  ALM_HVREL_FAIL_S : ArithShift  BitShiftNumber=7
  ALM_HVREL_FAIL_Sub : Subsystem
  ALM_HVREL_FAIL_sat : Saturate  UpperLimit=1  LowerLimit=0
  ALM_HVREL_FAILcv : DataTypeConversion
  ALM_LEAK_OC_Ad : Sum
  ALM_LEAK_OC_Convert : DataTypeConversion  OutDataTypeStr=uint32
  ALM_LEAK_OC_F : Gain
  ALM_LEAK_OC_L : simulink/Logic and Bit Operations/Bitwise Operator  logicop=AND  UseBitMask=on  BitMask=96  BitMaskRealWorld=Stored Integer
  ALM_LEAK_OC_O : Constant  Value=0  OutDataTypeStr=single
  ALM_LEAK_OC_S : ArithShift  BitShiftNumber=5
  ALM_LEAK_OC_Sub : Subsystem
  ALM_LEAK_OC_sat : Saturate  UpperLimit=3  LowerLimit=0
  ALM_LEAK_OCcv : DataTypeConversion
  ALM_PRECHRG_FAIL_Ad : Sum
  ALM_PRECHRG_FAIL_Convert : DataTypeConversion  OutDataTypeStr=uint32
  ALM_PRECHRG_FAIL_F : Gain
  ALM_PRECHRG_FAIL_L : simulink/Logic and Bit Operations/Bitwise Operator  logicop=AND  UseBitMask=on  BitMask=16  BitMaskRealWorld=Stored Integer
  ALM_PRECHRG_FAIL_O : Constant  Value=0  OutDataTypeStr=single
  ALM_PRECHRG_FAIL_S : ArithShift  BitShiftNumber=4
  ALM_PRECHRG_FAIL_Sub : Subsystem
  ALM_PRECHRG_FAIL_sat : Saturate  UpperLimit=1  LowerLimit=0
  ALM_PRECHRG_FAILcv : DataTypeConversion
  ALM_VCU_OFFLINE_Ad : Sum
  ALM_VCU_OFFLINE_Convert : DataTypeConversion  OutDataTypeStr=uint32
  ALM_VCU_OFFLINE_F : Gain
  ALM_VCU_OFFLINE_L : simulink/Logic and Bit Operations/Bitwise Operator  logicop=AND  UseBitMask=on  BitMask=3  BitMaskRealWorld=Stored Integer
  ALM_VCU_OFFLINE_O : Constant  Value=0  OutDataTypeStr=single
  ALM_VCU_OFFLINE_S : ArithShift
  ALM_VCU_OFFLINE_Sub : Subsystem
  ALM_VCU_OFFLINE_sat : Saturate  UpperLimit=3  LowerLimit=0
  ALM_VCU_OFFLINEcv : DataTypeConversion
  Demux : Demux  Outputs=8
  Terminator : Terminator
  Terminator1 : Terminator
  ALM_VCU_OFFLINE_Out : Outport
  ALM_PRECHRG_FAIL_Out : Outport  Port=2
  ALM_LEAK_OC_Out : Outport  Port=3
  ALM_HVREL_FAIL_Out : Outport  Port=4
  ALM_HALL_BREAK_Out : Outport  Port=5
  ALM_DSCH_OCT_Out : Outport  Port=6
  ALM_DSCH_OCS_Out : Outport  Port=7
  ALM_CHRG_OCT_Out : Outport  Port=8
  ALM_CHRG_OCS_Out : Outport  Port=9
  ALM_BSU_OFFLINE_Out : Outport  Port=10
  ALM_BSU_FAULT_Out : Outport  Port=11
  ALM_BMU_FAIL_Out : Outport  Port=12
  ALM_BATT_UC_Out : Outport  Port=13
  ALM_BATT_OC_Out : Outport  Port=14
  ALM_AUX_FAIL_Out : Outport  Port=15
  ALM_BATT_UV_Out : Outport  Port=16
  ALM_BATT_OV_Out : Outport  Port=17
  ALM_BATT_DT_Out : Outport  Port=18
  ALM_BATT_DV_Out : Outport  Port=19
  ALM_CELL_TBK_Out : Outport  Port=20
  ALM_CELL_IBK_Out : Outport  Port=21
  ALM_CELL_UT_Out : Outport  Port=22
  ALM_CELL_OT_Out : Outport  Port=23
  ALM_CELL_UV_Out : Outport  Port=24
  ALM_CELL_OV_Out : Outport  Port=25
  wires:
  ALM_VCU_OFFLINE_F/1 -> ALM_VCU_OFFLINE_Ad/1
  ALM_VCU_OFFLINE_O/1 -> ALM_VCU_OFFLINE_Ad/2
  ALM_VCU_OFFLINE_Ad/1 -> ALM_VCU_OFFLINE_sat/1
  ALM_VCU_OFFLINE_sat/1 -> ALM_VCU_OFFLINE_Out/1
  Demux/5 -> ALM_VCU_OFFLINE_Sub/1(In1), ALM_LEAK_OC_Sub/1(In1), ALM_BSU_FAULT_Sub/1(In1), ALM_BMU_FAIL_Sub/1(In1), ALM_AUX_FAIL_Sub/1(In1), ALM_PRECHRG_FAIL_Sub/1(In1)
  ALM_VCU_OFFLINE_Sub/1(Out1) -> ALM_VCU_OFFLINE_Convert/1
  ALM_VCU_OFFLINE_Convert/1 -> ALM_VCU_OFFLINE_L/1
  ALM_VCU_OFFLINE_L/1 -> ALM_VCU_OFFLINE_S/1
  ALM_VCU_OFFLINE_S/1 -> ALM_VCU_OFFLINEcv/1
  ALM_VCU_OFFLINEcv/1 -> ALM_VCU_OFFLINE_F/1
  ALM_PRECHRG_FAIL_F/1 -> ALM_PRECHRG_FAIL_Ad/1
  ALM_PRECHRG_FAIL_O/1 -> ALM_PRECHRG_FAIL_Ad/2
  ALM_PRECHRG_FAIL_Ad/1 -> ALM_PRECHRG_FAIL_sat/1
  ALM_PRECHRG_FAIL_sat/1 -> ALM_PRECHRG_FAIL_Out/1
  ALM_PRECHRG_FAIL_Sub/1(Out1) -> ALM_PRECHRG_FAIL_Convert/1
  ALM_PRECHRG_FAIL_Convert/1 -> ALM_PRECHRG_FAIL_L/1
  ALM_PRECHRG_FAIL_L/1 -> ALM_PRECHRG_FAIL_S/1
  ALM_PRECHRG_FAIL_S/1 -> ALM_PRECHRG_FAILcv/1
  ALM_PRECHRG_FAILcv/1 -> ALM_PRECHRG_FAIL_F/1
  ALM_LEAK_OC_F/1 -> ALM_LEAK_OC_Ad/1
  ALM_LEAK_OC_O/1 -> ALM_LEAK_OC_Ad/2
  ALM_LEAK_OC_Ad/1 -> ALM_LEAK_OC_sat/1
  ALM_LEAK_OC_sat/1 -> ALM_LEAK_OC_Out/1
  ALM_LEAK_OC_Sub/1(Out1) -> ALM_LEAK_OC_Convert/1
  ALM_LEAK_OC_Convert/1 -> ALM_LEAK_OC_L/1
  ALM_LEAK_OC_L/1 -> ALM_LEAK_OC_S/1
  ALM_LEAK_OC_S/1 -> ALM_LEAK_OCcv/1
  ALM_LEAK_OCcv/1 -> ALM_LEAK_OC_F/1
  ALM_HVREL_FAIL_F/1 -> ALM_HVREL_FAIL_Ad/1
  ALM_HVREL_FAIL_O/1 -> ALM_HVREL_FAIL_Ad/2
  ALM_HVREL_FAIL_Ad/1 -> ALM_HVREL_FAIL_sat/1
  ALM_HVREL_FAIL_sat/1 -> ALM_HVREL_FAIL_Out/1
  Demux/6 -> ALM_HVREL_FAIL_Sub/1(In1), ALM_HALL_BREAK_Sub/1(In1)
  ALM_HVREL_FAIL_Sub/1(Out1) -> ALM_HVREL_FAIL_Convert/1
  ALM_HVREL_FAIL_Convert/1 -> ALM_HVREL_FAIL_L/1
  ALM_HVREL_FAIL_L/1 -> ALM_HVREL_FAIL_S/1
  ALM_HVREL_FAIL_S/1 -> ALM_HVREL_FAILcv/1
  ALM_HVREL_FAILcv/1 -> ALM_HVREL_FAIL_F/1
  ALM_HALL_BREAK_F/1 -> ALM_HALL_BREAK_Ad/1
  ALM_HALL_BREAK_O/1 -> ALM_HALL_BREAK_Ad/2
  ALM_HALL_BREAK_Ad/1 -> ALM_HALL_BREAK_sat/1
  ALM_HALL_BREAK_sat/1 -> ALM_HALL_BREAK_Out/1
  ALM_HALL_BREAK_Sub/1(Out1) -> ALM_HALL_BREAK_Convert/1
  ALM_HALL_BREAK_Convert/1 -> ALM_HALL_BREAK_L/1
  ALM_HALL_BREAK_L/1 -> ALM_HALL_BREAK_S/1
  ALM_HALL_BREAK_S/1 -> ALM_HALL_BREAKcv/1
  ALM_HALL_BREAKcv/1 -> ALM_HALL_BREAK_F/1
  ALM_DSCH_OCT_F/1 -> ALM_DSCH_OCT_Ad/1
  ALM_DSCH_OCT_O/1 -> ALM_DSCH_OCT_Ad/2
  ALM_DSCH_OCT_Ad/1 -> ALM_DSCH_OCT_sat/1
  ALM_DSCH_OCT_sat/1 -> ALM_DSCH_OCT_Out/1
  Demux/4 -> ALM_DSCH_OCT_Sub/1(In1), ALM_DSCH_OCS_Sub/1(In1), ALM_CHRG_OCT_Sub/1(In1), ALM_BSU_OFFLINE_Sub/1(In1)
  ALM_DSCH_OCT_Sub/1(Out1) -> ALM_DSCH_OCT_Convert/1
  ALM_DSCH_OCT_Convert/1 -> ALM_DSCH_OCT_L/1
  ALM_DSCH_OCT_L/1 -> ALM_DSCH_OCT_S/1
  ALM_DSCH_OCT_S/1 -> ALM_DSCH_OCTcv/1
  ALM_DSCH_OCTcv/1 -> ALM_DSCH_OCT_F/1
  ALM_DSCH_OCS_F/1 -> ALM_DSCH_OCS_Ad/1
  ALM_DSCH_OCS_O/1 -> ALM_DSCH_OCS_Ad/2
  ALM_DSCH_OCS_Ad/1 -> ALM_DSCH_OCS_sat/1
  ALM_DSCH_OCS_sat/1 -> ALM_DSCH_OCS_Out/1
  ALM_DSCH_OCS_Sub/1(Out1) -> ALM_DSCH_OCS_Convert/1
  ALM_DSCH_OCS_Convert/1 -> ALM_DSCH_OCS_L/1
  ALM_DSCH_OCS_L/1 -> ALM_DSCH_OCS_S/1
  ALM_DSCH_OCS_S/1 -> ALM_DSCH_OCScv/1
  ALM_DSCH_OCScv/1 -> ALM_DSCH_OCS_F/1
  ALM_CHRG_OCT_F/1 -> ALM_CHRG_OCT_Ad/1
  ALM_CHRG_OCT_O/1 -> ALM_CHRG_OCT_Ad/2
  ALM_CHRG_OCT_Ad/1 -> ALM_CHRG_OCT_sat/1
  ALM_CHRG_OCT_sat/1 -> ALM_CHRG_OCT_Out/1
  ALM_CHRG_OCT_Sub/1(Out1) -> ALM_CHRG_OCT_Convert/1
  ALM_CHRG_OCT_Convert/1 -> ALM_CHRG_OCT_L/1
  ALM_CHRG_OCT_L/1 -> ALM_CHRG_OCT_S/1
  ALM_CHRG_OCT_S/1 -> ALM_CHRG_OCTcv/1
  ALM_CHRG_OCTcv/1 -> ALM_CHRG_OCT_F/1
  ALM_CHRG_OCS_F/1 -> ALM_CHRG_OCS_Ad/1
  ALM_CHRG_OCS_O/1 -> ALM_CHRG_OCS_Ad/2
  ALM_CHRG_OCS_Ad/1 -> ALM_CHRG_OCS_sat/1
  ALM_CHRG_OCS_sat/1 -> ALM_CHRG_OCS_Out/1
  Demux/3 -> ALM_BATT_OC_Sub/1(In1), ALM_BATT_UV_Sub/1(In1), ALM_BATT_UC_Sub/1(In1), ALM_CHRG_OCS_Sub/1(In1)
  ALM_CHRG_OCS_Sub/1(Out1) -> ALM_CHRG_OCS_Convert/1
  ALM_CHRG_OCS_Convert/1 -> ALM_CHRG_OCS_L/1
  ALM_CHRG_OCS_L/1 -> ALM_CHRG_OCS_S/1
  ALM_CHRG_OCS_S/1 -> ALM_CHRG_OCScv/1
  ALM_CHRG_OCScv/1 -> ALM_CHRG_OCS_F/1
  ALM_BSU_OFFLINE_F/1 -> ALM_BSU_OFFLINE_Ad/1
  ALM_BSU_OFFLINE_O/1 -> ALM_BSU_OFFLINE_Ad/2
  ALM_BSU_OFFLINE_Ad/1 -> ALM_BSU_OFFLINE_sat/1
  ALM_BSU_OFFLINE_sat/1 -> ALM_BSU_OFFLINE_Out/1
  ALM_BSU_OFFLINE_Sub/1(Out1) -> ALM_BSU_OFFLINE_Convert/1
  ALM_BSU_OFFLINE_Convert/1 -> ALM_BSU_OFFLINE_L/1
  ALM_BSU_OFFLINE_L/1 -> ALM_BSU_OFFLINE_S/1
  ALM_BSU_OFFLINE_S/1 -> ALM_BSU_OFFLINEcv/1
  ALM_BSU_OFFLINEcv/1 -> ALM_BSU_OFFLINE_F/1
  ALM_BSU_FAULT_F/1 -> ALM_BSU_FAULT_Ad/1
  ALM_BSU_FAULT_O/1 -> ALM_BSU_FAULT_Ad/2
  ALM_BSU_FAULT_Ad/1 -> ALM_BSU_FAULT_sat/1
  ALM_BSU_FAULT_sat/1 -> ALM_BSU_FAULT_Out/1
  ALM_BSU_FAULT_Sub/1(Out1) -> ALM_BSU_FAULT_Convert/1
  ALM_BSU_FAULT_Convert/1 -> ALM_BSU_FAULT_L/1
  ALM_BSU_FAULT_L/1 -> ALM_BSU_FAULT_S/1
  ALM_BSU_FAULT_S/1 -> ALM_BSU_FAULTcv/1
  ALM_BSU_FAULTcv/1 -> ALM_BSU_FAULT_F/1
  ALM_BMU_FAIL_F/1 -> ALM_BMU_FAIL_Ad/1
  ALM_BMU_FAIL_O/1 -> ALM_BMU_FAIL_Ad/2
  ALM_BMU_FAIL_Ad/1 -> ALM_BMU_FAIL_sat/1
  ALM_BMU_FAIL_sat/1 -> ALM_BMU_FAIL_Out/1
  ALM_BMU_FAIL_Sub/1(Out1) -> ALM_BMU_FAIL_Convert/1
  ALM_BMU_FAIL_Convert/1 -> ALM_BMU_FAIL_L/1
  ALM_BMU_FAIL_L/1 -> ALM_BMU_FAIL_S/1
  ALM_BMU_FAIL_S/1 -> ALM_BMU_FAILcv/1
  ALM_BMU_FAILcv/1 -> ALM_BMU_FAIL_F/1
  ALM_BATT_UC_F/1 -> ALM_BATT_UC_Ad/1
  ALM_BATT_UC_O/1 -> ALM_BATT_UC_Ad/2
  ALM_BATT_UC_Ad/1 -> ALM_BATT_UC_sat/1
  ALM_BATT_UC_sat/1 -> ALM_BATT_UC_Out/1
  ALM_BATT_UC_Sub/1(Out1) -> ALM_BATT_UC_Convert/1
  ALM_BATT_UC_Convert/1 -> ALM_BATT_UC_L/1
  ALM_BATT_UC_L/1 -> ALM_BATT_UC_S/1
  ALM_BATT_UC_S/1 -> ALM_BATT_UCcv/1
  ALM_BATT_UCcv/1 -> ALM_BATT_UC_F/1
  ALM_BATT_OC_F/1 -> ALM_BATT_OC_Ad/1
  ALM_BATT_OC_O/1 -> ALM_BATT_OC_Ad/2
  ALM_BATT_OC_Ad/1 -> ALM_BATT_OC_sat/1
  ALM_BATT_OC_sat/1 -> ALM_BATT_OC_Out/1
  ALM_BATT_OC_Sub/1(Out1) -> ALM_BATT_OC_Convert/1
  ALM_BATT_OC_Convert/1 -> ALM_BATT_OC_L/1
  ALM_BATT_OC_L/1 -> ALM_BATT_OC_S/1
  ALM_BATT_OC_S/1 -> ALM_BATT_OCcv/1
  ALM_BATT_OCcv/1 -> ALM_BATT_OC_F/1
  ALM_AUX_FAIL_F/1 -> ALM_AUX_FAIL_Ad/1
  ALM_AUX_FAIL_O/1 -> ALM_AUX_FAIL_Ad/2
  ALM_AUX_FAIL_Ad/1 -> ALM_AUX_FAIL_sat/1
  ALM_AUX_FAIL_sat/1 -> ALM_AUX_FAIL_Out/1
  ALM_AUX_FAIL_Sub/1(Out1) -> ALM_AUX_FAIL_Convert/1
  ALM_AUX_FAIL_Convert/1 -> ALM_AUX_FAIL_L/1
  ALM_AUX_FAIL_L/1 -> ALM_AUX_FAIL_S/1
  ALM_AUX_FAIL_S/1 -> ALM_AUX_FAILcv/1
  ALM_AUX_FAILcv/1 -> ALM_AUX_FAIL_F/1
  ALM_BATT_UV_F/1 -> ALM_BATT_UV_Ad/1
  ALM_BATT_UV_O/1 -> ALM_BATT_UV_Ad/2
  ALM_BATT_UV_Ad/1 -> ALM_BATT_UV_sat/1
  ALM_BATT_UV_sat/1 -> ALM_BATT_UV_Out/1
  ALM_BATT_UV_Sub/1(Out1) -> ALM_BATT_UV_Convert/1
  ALM_BATT_UV_Convert/1 -> ALM_BATT_UV_L/1
  ALM_BATT_UV_L/1 -> ALM_BATT_UV_S/1
  ALM_BATT_UV_S/1 -> ALM_BATT_UVcv/1
  ALM_BATT_UVcv/1 -> ALM_BATT_UV_F/1
  ALM_BATT_OV_F/1 -> ALM_BATT_OV_Ad/1
  ALM_BATT_OV_O/1 -> ALM_BATT_OV_Ad/2
  ALM_BATT_OV_Ad/1 -> ALM_BATT_OV_sat/1
  ALM_BATT_OV_sat/1 -> ALM_BATT_OV_Out/1
  Demux/2 -> ALM_CELL_TBK_Sub/1(In1), ALM_CELL_IBK_Sub/1(In1), ALM_BATT_DV_Sub/1(In1), ALM_BATT_DT_Sub/1(In1), ALM_BATT_OV_Sub/1(In1)
  ALM_BATT_OV_Sub/1(Out1) -> ALM_BATT_OV_Convert/1
  ALM_BATT_OV_Convert/1 -> ALM_BATT_OV_L/1
  ALM_BATT_OV_L/1 -> ALM_BATT_OV_S/1
  ALM_BATT_OV_S/1 -> ALM_BATT_OVcv/1
  ALM_BATT_OVcv/1 -> ALM_BATT_OV_F/1
  ALM_BATT_DT_F/1 -> ALM_BATT_DT_Ad/1
  ALM_BATT_DT_O/1 -> ALM_BATT_DT_Ad/2
  ALM_BATT_DT_Ad/1 -> ALM_BATT_DT_sat/1
  ALM_BATT_DT_sat/1 -> ALM_BATT_DT_Out/1
  ALM_BATT_DT_Sub/1(Out1) -> ALM_BATT_DT_Convert/1
  ALM_BATT_DT_Convert/1 -> ALM_BATT_DT_L/1
  ALM_BATT_DT_L/1 -> ALM_BATT_DT_S/1
  ALM_BATT_DT_S/1 -> ALM_BATT_DTcv/1
  ALM_BATT_DTcv/1 -> ALM_BATT_DT_F/1
  ALM_BATT_DV_F/1 -> ALM_BATT_DV_Ad/1
  ALM_BATT_DV_O/1 -> ALM_BATT_DV_Ad/2
  ALM_BATT_DV_Ad/1 -> ALM_BATT_DV_sat/1
  ALM_BATT_DV_sat/1 -> ALM_BATT_DV_Out/1
  ALM_BATT_DV_Sub/1(Out1) -> ALM_BATT_DV_Convert/1
  ALM_BATT_DV_Convert/1 -> ALM_BATT_DV_L/1
  ALM_BATT_DV_L/1 -> ALM_BATT_DV_S/1
  ALM_BATT_DV_S/1 -> ALM_BATT_DVcv/1
  ALM_BATT_DVcv/1 -> ALM_BATT_DV_F/1
  ALM_CELL_TBK_F/1 -> ALM_CELL_TBK_Ad/1
  ALM_CELL_TBK_O/1 -> ALM_CELL_TBK_Ad/2
  ALM_CELL_TBK_Ad/1 -> ALM_CELL_TBK_sat/1
  ALM_CELL_TBK_sat/1 -> ALM_CELL_TBK_Out/1
  ALM_CELL_TBK_Sub/1(Out1) -> ALM_CELL_TBK_Convert/1
  ALM_CELL_TBK_Convert/1 -> ALM_CELL_TBK_L/1
  ALM_CELL_TBK_L/1 -> ALM_CELL_TBK_S/1
  ALM_CELL_TBK_S/1 -> ALM_CELL_TBKcv/1
  ALM_CELL_TBKcv/1 -> ALM_CELL_TBK_F/1
  ALM_CELL_IBK_F/1 -> ALM_CELL_IBK_Ad/1
  ALM_CELL_IBK_O/1 -> ALM_CELL_IBK_Ad/2
  ALM_CELL_IBK_Ad/1 -> ALM_CELL_IBK_sat/1
  ALM_CELL_IBK_sat/1 -> ALM_CELL_IBK_Out/1
  ALM_CELL_IBK_Sub/1(Out1) -> ALM_CELL_IBK_Convert/1
  ALM_CELL_IBK_Convert/1 -> ALM_CELL_IBK_L/1
  ALM_CELL_IBK_L/1 -> ALM_CELL_IBK_S/1
  ALM_CELL_IBK_S/1 -> ALM_CELL_IBKcv/1
  ALM_CELL_IBKcv/1 -> ALM_CELL_IBK_F/1
  ALM_CELL_UT_F/1 -> ALM_CELL_UT_Ad/1
  ALM_CELL_UT_O/1 -> ALM_CELL_UT_Ad/2
  ALM_CELL_UT_Ad/1 -> ALM_CELL_UT_sat/1
  ALM_CELL_UT_sat/1 -> ALM_CELL_UT_Out/1
  Demux/1 -> ALM_CELL_UV_Sub/1(In1), ALM_CELL_OV_Sub/1(In1), ALM_CELL_OT_Sub/1(In1), ALM_CELL_UT_Sub/1(In1)
  ALM_CELL_UT_Sub/1(Out1) -> ALM_CELL_UT_Convert/1
  ALM_CELL_UT_Convert/1 -> ALM_CELL_UT_L/1
  ALM_CELL_UT_L/1 -> ALM_CELL_UT_S/1
  ALM_CELL_UT_S/1 -> ALM_CELL_UTcv/1
  ALM_CELL_UTcv/1 -> ALM_CELL_UT_F/1
  ALM_CELL_OT_F/1 -> ALM_CELL_OT_Ad/1
  ALM_CELL_OT_O/1 -> ALM_CELL_OT_Ad/2
  ALM_CELL_OT_Ad/1 -> ALM_CELL_OT_sat/1
  ALM_CELL_OT_sat/1 -> ALM_CELL_OT_Out/1
  ALM_CELL_OT_Sub/1(Out1) -> ALM_CELL_OT_Convert/1
  ALM_CELL_OT_Convert/1 -> ALM_CELL_OT_L/1
  ALM_CELL_OT_L/1 -> ALM_CELL_OT_S/1
  ALM_CELL_OT_S/1 -> ALM_CELL_OTcv/1
  ALM_CELL_OTcv/1 -> ALM_CELL_OT_F/1
  ALM_CELL_UV_F/1 -> ALM_CELL_UV_Ad/1
  ALM_CELL_UV_O/1 -> ALM_CELL_UV_Ad/2
  ALM_CELL_UV_Ad/1 -> ALM_CELL_UV_sat/1
  ALM_CELL_UV_sat/1 -> ALM_CELL_UV_Out/1
  ALM_CELL_UV_Sub/1(Out1) -> ALM_CELL_UV_Convert/1
  ALM_CELL_UV_Convert/1 -> ALM_CELL_UV_L/1
  ALM_CELL_UV_L/1 -> ALM_CELL_UV_S/1
  ALM_CELL_UV_S/1 -> ALM_CELL_UVcv/1
  ALM_CELL_UVcv/1 -> ALM_CELL_UV_F/1
  ALM_CELL_OV_F/1 -> ALM_CELL_OV_Ad/1
  ALM_CELL_OV_O/1 -> ALM_CELL_OV_Ad/2
  ALM_CELL_OV_Ad/1 -> ALM_CELL_OV_sat/1
  ALM_CELL_OV_sat/1 -> ALM_CELL_OV_Out/1
  ALM_CELL_OV_Sub/1(Out1) -> ALM_CELL_OV_Convert/1
  ALM_CELL_OV_Convert/1 -> ALM_CELL_OV_L/1
  ALM_CELL_OV_L/1 -> ALM_CELL_OV_S/1
  ALM_CELL_OV_S/1 -> ALM_CELL_OVcv/1
  ALM_CELL_OVcv/1 -> ALM_CELL_OV_F/1
  input/1 -> Demux/1
  Demux/7 -> Terminator/1
  Demux/8 -> Terminator1/1

== system FSAC2021_V1_Running/VCU_CAN_Read/PCANB(BMS、DRIVE_MOTOR)/BMS_HCU_MAXT1/CoolingCtl_Sub ==
  In1 : Inport
  Out1 : Outport
  wires:
  In1/1 -> Out1/1

== system FSAC2021_V1_Running/VCU_CAN_Read/PCANB(BMS、DRIVE_MOTOR)/BMS_HCU_MAXT1/HeatingCtl_Sub ==
  In1 : Inport
  Out1 : Outport
  wires:
  In1/1 -> Out1/1

== system FSAC2021_V1_Running/VCU_CAN_Read/PCANB(BMS、DRIVE_MOTOR)/BMS_HCU_MAXT1/MaxTempNo_Sub ==
  In1 : Inport
  Out1 : Outport
  wires:
  In1/1 -> Out1/1

== system FSAC2021_V1_Running/VCU_CAN_Read/PCANB(BMS、DRIVE_MOTOR)/BMS_HCU_MAXT1/MaxTemp_Sub ==
  In1 : Inport
  Out1 : Outport
  wires:
  In1/1 -> Out1/1

== system FSAC2021_V1_Running/VCU_CAN_Read/PCANB(BMS、DRIVE_MOTOR)/BMS_HCU_MAXT1/MinTempNo_Sub ==
  In1 : Inport
  Out1 : Outport
  wires:
  In1/1 -> Out1/1

== system FSAC2021_V1_Running/VCU_CAN_Read/PCANB(BMS、DRIVE_MOTOR)/BMS_HCU_MAXT1/MinTemp_Sub ==
  In1 : Inport
  Out1 : Outport
  wires:
  In1/1 -> Out1/1
